simulink model "trim_temp"  (R2021b)
settings: Solver=VariableStepAuto  StartTime=0.0  StopTime=10.0  RelTol=1e-3
undefined symbols (not defined in the file or in its folder): h0, RCAM_model, u1max, u1min, u2max, u2min, u3max, u3min, u4max, u4min, uo, x0
settings Model: Creator=khanh  LastModifiedBy=khanh

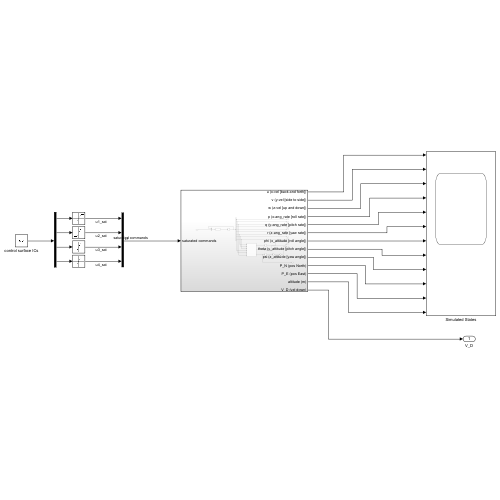
[thumbnail: Simulink's stored preview of the top-level diagram]
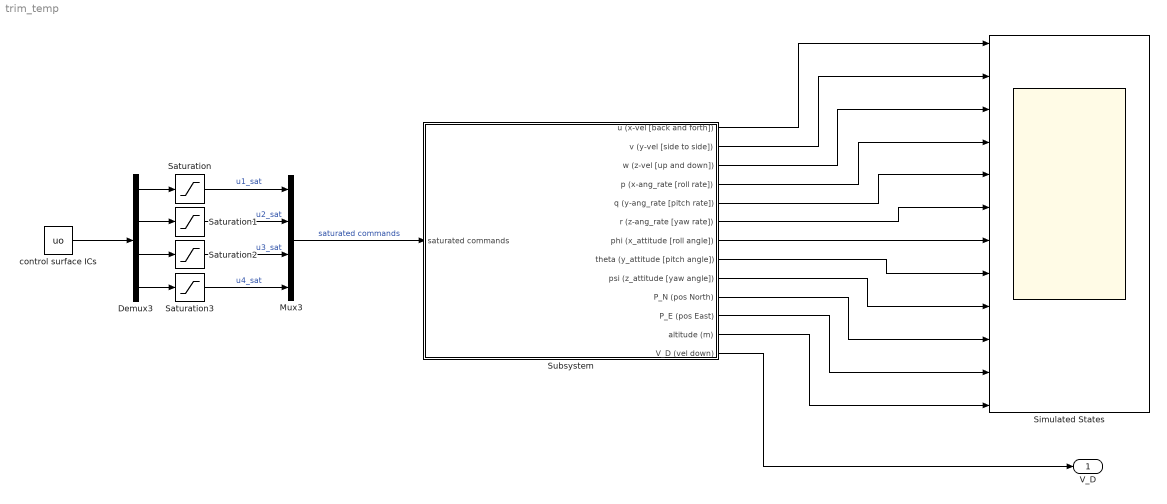
== system trim_temp ==
  Demux3 : Demux
  Mux3 : Mux
  Saturation : Saturate  UpperLimit=u1max  LowerLimit=u1min
  Saturation1 : Saturate  UpperLimit=u2max  LowerLimit=u2min
  Saturation2 : Saturate  UpperLimit=u3max  LowerLimit=u3min
  Saturation3 : Saturate  UpperLimit=u4max  LowerLimit=u4min
  Simulated States : Scope  NumInputPorts=12
  Subsystem : Subsystem
  control surface ICs : Constant  Value=uo
  V_D : Outport
  wires:
  Demux3/1 -> Saturation/1
  Saturation1/1 -> Mux3/2  "u2_sat"
  Demux3/3 -> Saturation2/1
  control surface ICs/1 -> Demux3/1
  Demux3/2 -> Saturation1/1
  Demux3/4 -> Saturation3/1
  Saturation/1 -> Mux3/1  "u1_sat"
  Saturation3/1 -> Mux3/4  "u4_sat"
  Saturation2/1 -> Mux3/3  "u3_sat"
  Mux3/1 -> Subsystem/1(saturated commands)  "saturated commands"
  Subsystem/1(u (x-vel [back and forth])) -> Simulated States/1
  Subsystem/2(v (y-vel [side to side])) -> Simulated States/2
  Subsystem/3(w (z-vel [up and down])) -> Simulated States/3
  Subsystem/4(p (x-ang_rate [roll rate])) -> Simulated States/4
  Subsystem/5(q (y-ang_rate [pitch rate])) -> Simulated States/5
  Subsystem/6(r (z-ang_rate [yaw rate])) -> Simulated States/6
  Subsystem/7(phi (x_attitude [roll angle])) -> Simulated States/7
  Subsystem/8(theta (y_attitude [pitch angle])) -> Simulated States/8
  Subsystem/9(psi (z_attitude [yaw angle])) -> Simulated States/9
  Subsystem/10(P_N (pos North)) -> Simulated States/10
  Subsystem/11(P_E (pos East)) -> Simulated States/11
  Subsystem/12(altitude (m)) -> Simulated States/12
  Subsystem/13(V_D (vel down)) -> V_D/1

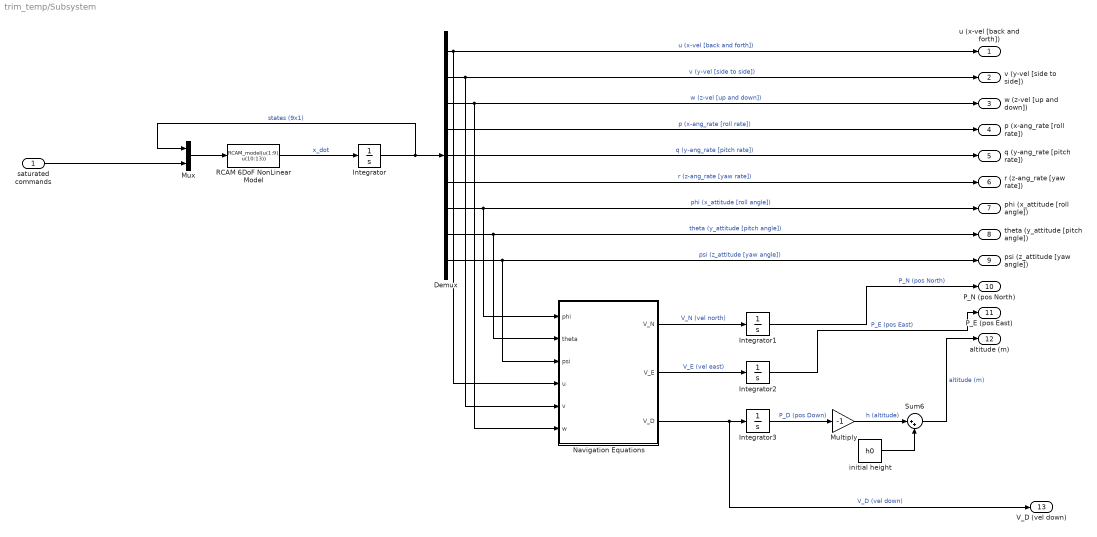
== system trim_temp/Subsystem ==
  saturated commands : Inport
  Demux : Demux  Outputs=9
  Integrator : Integrator  InitialCondition=x0
  Integrator1 : Integrator
  Integrator2 : Integrator
  Integrator3 : Integrator
  Multiply : Gain  Gain=-1
  Mux : Mux  Inputs=2
  Navigation Equations : MATLAB Function  TreatAsAtomicUnit=on
  RCAM 6DoF NonLinear Model : MATLABFcn  MATLABFcn=RCAM_model(u(1:9), u(10:13))
  Sum6 : Sum  Inputs=|++
  initial height : Constant  Value=h0
  u (x-vel [back and forth]) : Outport
  v (y-vel [side to side]) : Outport  Port=2
  w (z-vel [up and down]) : Outport  Port=3
  p (x-ang_rate [roll rate]) : Outport  Port=4
  q (y-ang_rate [pitch rate]) : Outport  Port=5
  r (z-ang_rate [yaw rate]) : Outport  Port=6
  phi (x_attitude [roll angle]) : Outport  Port=7
  theta (y_attitude [pitch angle]) : Outport  Port=8
  psi (z_attitude [yaw angle]) : Outport  Port=9
  P_N (pos North) : Outport  Port=10
  P_E (pos East) : Outport  Port=11
  altitude (m) : Outport  Port=12
  V_D (vel down) : Outport  Port=13
  wires:
  Integrator3/1 -> Multiply/1  "P_D (pos Down)"
  Multiply/1 -> Sum6/1  "h (altitude)"
  Navigation Equations/3(V_D) -> V_D (vel down)/1, Integrator3/1  "V_D (vel down)"
  Demux/3 -> w (z-vel [up and down])/1, Navigation Equations/6(w)  "w (z-vel [up and down])"
  Navigation Equations/1(V_N) -> Integrator1/1  "V_N (vel north)"
  initial height/1 -> Sum6/2
  Demux/1 -> u (x-vel [back and forth])/1, Navigation Equations/4(u)  "u (x-vel [back and forth])"
  Demux/7 -> phi (x_attitude [roll angle])/1, Navigation Equations/1(phi)  "phi (x_attitude [roll angle])"
  RCAM 6DoF NonLinear Model/1 -> Integrator/1  "x_dot"
  Demux/8 -> theta (y_attitude [pitch angle])/1, Navigation Equations/2(theta)  "theta (y_attitude [pitch angle])"
  Demux/4 -> p (x-ang_rate [roll rate])/1  "p (x-ang_rate [roll rate])"
  Navigation Equations/2(V_E) -> Integrator2/1  "V_E (vel east)"
  Mux/1 -> RCAM 6DoF NonLinear Model/1
  Integrator/1 -> Mux/1, Demux/1  "states (9x1)"
  Demux/9 -> psi (z_attitude [yaw angle])/1, Navigation Equations/3(psi)  "psi (z_attitude [yaw angle])"
  Demux/2 -> v (y-vel [side to side])/1, Navigation Equations/5(v)  "v (y-vel [side to side])"
  Demux/6 -> r (z-ang_rate [yaw rate])/1  "r (z-ang_rate [yaw rate])"
  Demux/5 -> q (y-ang_rate [pitch rate])/1  "q (y-ang_rate [pitch rate])"
  Integrator1/1 -> P_N (pos North)/1  "P_N (pos North)"
  saturated commands/1 -> Mux/2
  Sum6/1 -> altitude (m)/1  "altitude (m)"
  Integrator2/1 -> P_E (pos East)/1  "P_E (pos East)"

== matlab function trim_temp/Subsystem/Navigation Equations ==
  data: phi input; theta input; psi input; u input; V_N output; v input; w input; V_E output; V_D output
function [V_N, V_E, V_D] = navigation_equation(phi, theta, psi, u, v, w)

x7 = phi;
x8 = theta;
x9 = psi;
x1 = u;
x2 = v;
x3 = w;

V_b = [x1; x2; x3];

%navigation equations
C1v = [cos(x9) sin(x9) 0; -sin(x9) cos(x9) 0; 0 0 1];

C21 = [cos(x8) 0 -sin(x8); 0 1 0; sin(x8) 0 cos(x8)];

Cb2 = [1 0 0; 0 cos(x7) sin(x7); 0 -sin(x7) cos(x7)];

Cvb = Cb2*C21*C1v;
Cvb = Cvb';

vel_vector = Cvb*V_b;

V_N = vel_vector(1);
V_E = vel_vector(2);
V_D = vel_vector(3);

end
